simulink model "time_delay"  (R2021a)
settings: Solver=ode23t  StartTime=0.0  StopTime=20.0  RelTol=1e-3
settings Model: Creator=Suman  LastModifiedBy=Suman

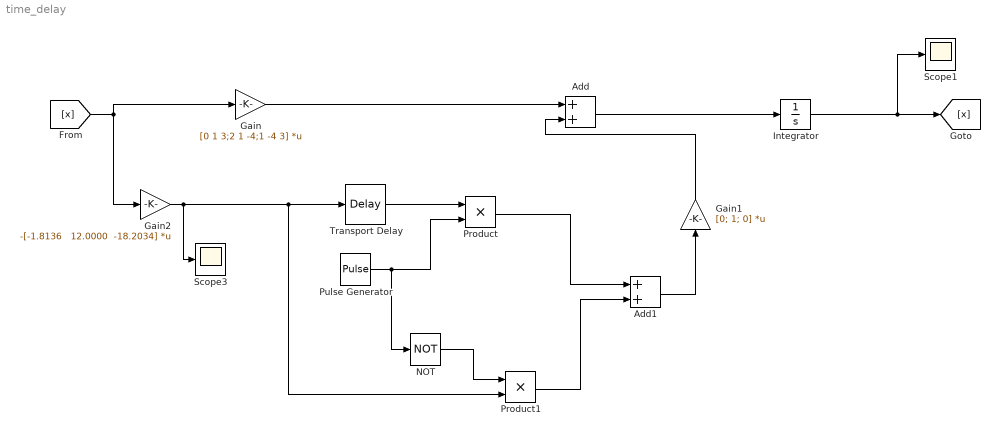
== system time_delay ==
  Add : Sum
  Add1 : Sum
  Gain : Gain  Gain=[0 1 3;2 1 -4;1 -4 3]  Multiplication=Matrix(K*u) (u vector)
  Gain1 : Gain  Gain=[0; 1; 0]  Multiplication=Matrix(K*u)
  Gain2 : Gain  Gain="-[-1.8136   12.0000  -18.2034]"  Multiplication=Matrix(K*u) (u vector)
  Integrator : Integrator  InitialCondition=[2;3;1]
  NOT : Logic  Operator=NOT  IconShape=distinctive  AllPortsSameDT=off  OutDataTypeStr=boolean
  Product : Product
  Product1 : Product
  Pulse Generator : DiscretePulseGenerator  PulseType=Time based  Period=20  PulseWidth=10  PhaseDelay=3
  Scope1 : Scope
  Scope3 : Scope
  Transport Delay : TransportDelay  DelayTime=0.5
  wires:
  Integrator/1 -> Scope1/1, [x]
  [x] -> Gain2/1, Gain/1
  Gain/1 -> Add/1
  Add/1 -> Integrator/1
  Gain2/1 -> Product1/2, Transport Delay/1, Scope3/1
  Transport Delay/1 -> Product/1
  Pulse Generator/1 -> NOT/1, Product/2
  NOT/1 -> Product1/1
  Product/1 -> Add1/1
  Product1/1 -> Add1/2
  Add1/1 -> Gain1/1
  Gain1/1 -> Add/2
